simulink model "fizzbuzz"  (R2017a)
settings: Solver=VariableStepAuto  StartTime=0.0  StopTime=31.0  RelTol=1e-3
libraries: simulink x5, dspswit3 x1
settings Model: Creator=reyesc  LastModifiedBy=reyesc

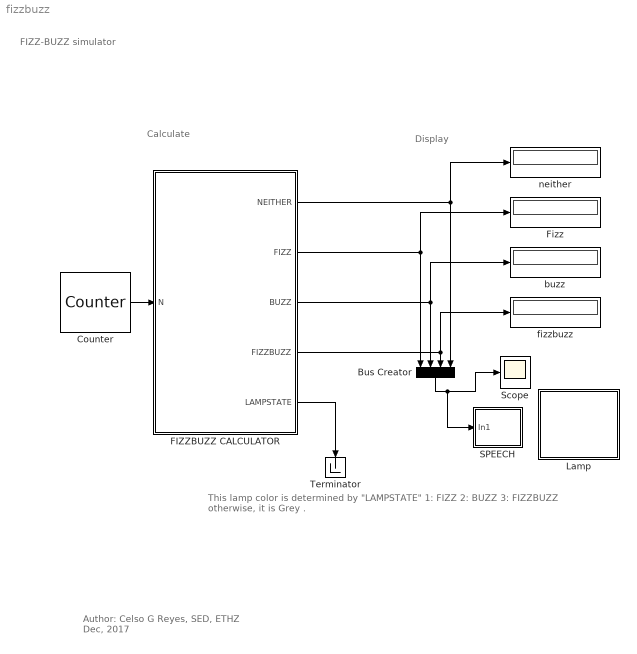
== system fizzbuzz ==
  note: Display
  note: Calculate
  note: This lamp color is determined by "LAMPSTATE"
      |
      | 1: FIZZ
      | 2: BUZZ
      | 3: FIZZBUZZ
      |
      | otherwise, it is Grey .
  note: Author: Celso G Reyes, SED, ETHZ
      | Dec, 2017
  note: FIZZ-BUZZ simulator
  Bus Creator : BusCreator  Inputs=4
  Counter : dspswit3/Counter  Direction=Up  CountEvent=Free running  CounterSize=User defined  MaxCount=100  InitialCount=0  Output=Count  HitValue=32  ResetInput=on  SamplesPerFrame=1  Ts=1  CntDtype=double  HitDtype=Logical
  FIZZBUZZ CALCULATOR : Subsystem
  Fizz : Display
  Lamp : Subsystem  DialogController=hmiCreateDDGDialog  IsWebBlock=on  mask(MWDashboardBlock){webBlockId=59f860f3-1faa-406f-b880-97fe9cd8e32d, webBlockType=lamp, ShowInLibBrowser=on, ShowInitialText=on, HMISrcModelName=fizzbuzz_simulator_c}
      mask prompts: webBlockType "WebBlock Type"; HMISrcModelName "Source Model"
      mask help: SimulinkHMI:dialogs:LampDialogDesc
      mask Help: helpview([docroot '/mapfiles/simulink.map'], 'hmi_lamp')
      mask Display:
      | if strcmp(get_param(bdroot(gcb),'BlockDiagramType'), 'library')
      |     image([(matlabroot) '/toolbox/simulink/hmi/icons/Lamp.png']);
      | end
  SPEECH : Subsystem
  Scope : Scope
  Terminator : Terminator
  buzz : Display
  fizzbuzz : Display
  neither : Display
  wires:
  Bus Creator/1 -> SPEECH/1(In1), Scope/1
  FIZZBUZZ CALCULATOR/4(FIZZBUZZ) -> fizzbuzz/1, Bus Creator/3
  FIZZBUZZ CALCULATOR/3(BUZZ) -> buzz/1, Bus Creator/2
  FIZZBUZZ CALCULATOR/2(FIZZ) -> Fizz/1, Bus Creator/1
  FIZZBUZZ CALCULATOR/1(NEITHER) -> neither/1, Bus Creator/4
  Counter/1 -> FIZZBUZZ CALCULATOR/1(N)
  FIZZBUZZ CALCULATOR/5(LAMPSTATE) -> Terminator/1

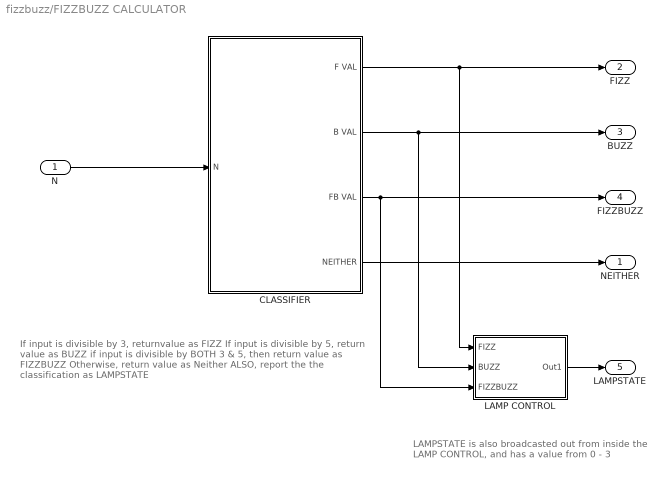
== system fizzbuzz/FIZZBUZZ CALCULATOR ==
  note: If input is divisible by 3, returnvalue as FIZZ
      |
      | If input is divisible by 5, return value as BUZZ
      |
      | if input is divisible by BOTH 3 & 5, then
      | return value as FIZZBUZZ
      |
      | Otherwise, return value as Neither
      |
      | ALSO, report the the classification as LAMPSTATE
  note: LAMPSTATE is also broadcasted out from inside
      | the LAMP CONTROL, and has a value from 0 - 3
  N : Inport
  CLASSIFIER : Subsystem
  LAMP CONTROL : Subsystem
  NEITHER : Outport
  FIZZ : Outport  Port=2
  BUZZ : Outport  Port=3
  FIZZBUZZ : Outport  Port=4
  LAMPSTATE : Outport  Port=5
  wires:
  LAMP CONTROL/1(Out1) -> LAMPSTATE/1
  N/1 -> CLASSIFIER/1(N)
  CLASSIFIER/4(NEITHER) -> NEITHER/1
  CLASSIFIER/3(FB VAL) -> LAMP CONTROL/3(FIZZBUZZ), FIZZBUZZ/1
  CLASSIFIER/1(F VAL) -> FIZZ/1, LAMP CONTROL/1(FIZZ)
  CLASSIFIER/2(B VAL) -> BUZZ/1, LAMP CONTROL/2(BUZZ)

== system fizzbuzz/Lamp ==

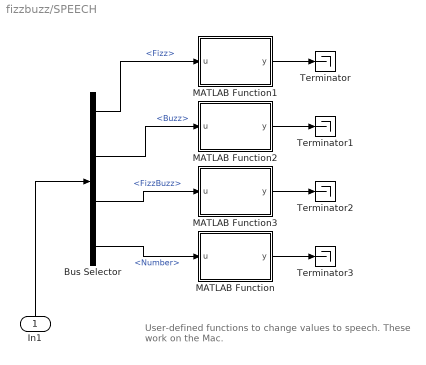
== system fizzbuzz/SPEECH ==
  note: User-defined functions to change values to speech.
      | These work on the Mac.
  In1 : Inport
  Bus Selector : BusSelector  OutputSignals=Fizz,Buzz,FizzBuzz,Number
  MATLAB Function : MATLAB Function  TreatAsAtomicUnit=on
  MATLAB Function1 : MATLAB Function  TreatAsAtomicUnit=on
  MATLAB Function2 : MATLAB Function  TreatAsAtomicUnit=on
  MATLAB Function3 : MATLAB Function  TreatAsAtomicUnit=on
  Terminator{,1..3} (4 alike) : Terminator
  wires:
  In1/1 -> Bus Selector/1
  Bus Selector/2 -> MATLAB Function2/1(u)  "<Buzz>"
  MATLAB Function2/1(y) -> Terminator1/1
  MATLAB Function3/1(y) -> Terminator2/1
  MATLAB Function1/1(y) -> Terminator/1
  Bus Selector/1 -> MATLAB Function1/1(u)  "<Fizz>"
  Bus Selector/4 -> MATLAB Function/1(u)  "<Number>"
  Bus Selector/3 -> MATLAB Function3/1(u)  "<FizzBuzz>"
  MATLAB Function/1(y) -> Terminator3/1

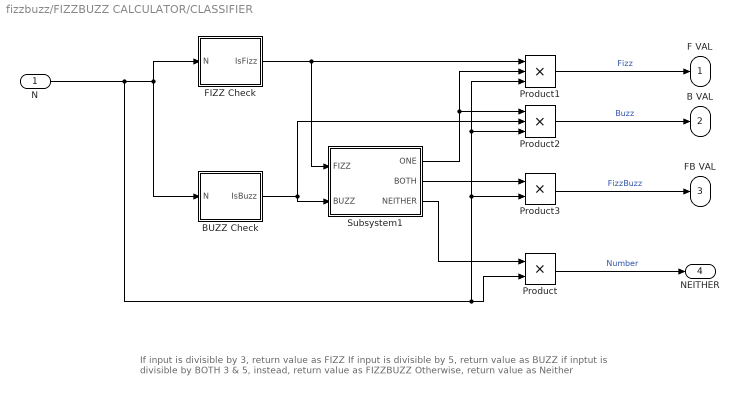
== system fizzbuzz/FIZZBUZZ CALCULATOR/CLASSIFIER ==
  note: If input is divisible by 3, return value as FIZZ
      | If input is divisible by 5, return value as BUZZ
      | if inptut is divisible by BOTH 3 & 5, instead, return value as FIZZBUZZ
      | Otherwise, return value as Neither
  N : Inport
  BUZZ Check : Subsystem
  FIZZ Check : Subsystem
  Product : Product
  Product1 : Product  Inputs=3
  Product2 : Product  Inputs=3
  Product3 : Product
  Subsystem1 : Subsystem
  F VAL : Outport
  B VAL : Outport  Port=2
  FB VAL : Outport  Port=3
  NEITHER : Outport  Port=4
  wires:
  Product1/1 -> F VAL/1  "Fizz"
  Product3/1 -> FB VAL/1  "FizzBuzz"
  Product/1 -> NEITHER/1  "Number"
  N/1 -> Product3/2, Product1/3, Product2/3, Product/2, BUZZ Check/1(N), FIZZ Check/1(N)
  Product2/1 -> B VAL/1  "Buzz"
  BUZZ Check/1(IsBuzz) -> Subsystem1/2(BUZZ), Product2/2
  FIZZ Check/1(IsFizz) -> Product1/1, Subsystem1/1(FIZZ)
  Subsystem1/2(BOTH) -> Product3/1
  Subsystem1/3(NEITHER) -> Product/1
  Subsystem1/1(ONE) -> Product1/2, Product2/1

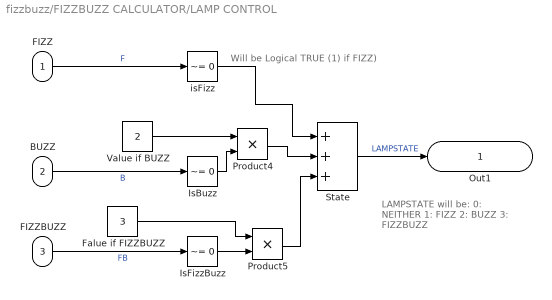
== system fizzbuzz/FIZZBUZZ CALCULATOR/LAMP CONTROL ==
  note: Will be Logical TRUE (1) if FIZZ)
  note: LAMPSTATE will be:
      |
      | 0: NEITHER
      | 1: FIZZ
      | 2: BUZZ
      | 3: FIZZBUZZ
  FIZZ : Inport
  BUZZ : Inport  Port=2
  FIZZBUZZ : Inport  Port=3
  Falue if FIZZBUZZ : Constant  Value=3
  IsBuzz : simulink/Logic and Bit Operations/Compare To Zero  relop=~=  OutDataTypeStr=boolean
  IsFizzBuzz : simulink/Logic and Bit Operations/Compare To Zero  relop=~=  OutDataTypeStr=boolean
  Product4 : Product
  Product5 : Product
  State : Sum  Inputs=+++
  Value if BUZZ : Constant  Value=2
  isFizz : simulink/Logic and Bit Operations/Compare To Zero  relop=~=  OutDataTypeStr=boolean
  Out1 : Outport
  wires:
  IsFizzBuzz/1 -> Product5/2
  isFizz/1 -> State/1
  Product4/1 -> State/2
  IsBuzz/1 -> Product4/2
  Product5/1 -> State/3
  Falue if FIZZBUZZ/1 -> Product5/1
  Value if BUZZ/1 -> Product4/1
  State/1 -> Out1/1  "LAMPSTATE"
  FIZZ/1 -> isFizz/1  "F"
  BUZZ/1 -> IsBuzz/1  "B"
  FIZZBUZZ/1 -> IsFizzBuzz/1  "FB"

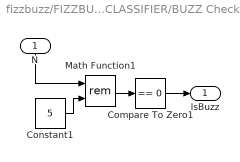
== system fizzbuzz/FIZZBUZZ CALCULATOR/CLASSIFIER/BUZZ Check ==
  N : Inport
  Compare To Zero1 : simulink/Logic and Bit Operations/Compare To Zero  relop===  OutDataTypeStr=boolean
  Constant1 : Constant  Value=5
  Math Function1 : Math  Operator=rem  SaturateOnIntegerOverflow=on
  IsBuzz : Outport
  wires:
  Constant1/1 -> Math Function1/2
  Math Function1/1 -> Compare To Zero1/1
  Compare To Zero1/1 -> IsBuzz/1
  N/1 -> Math Function1/1

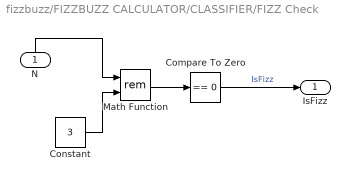
== system fizzbuzz/FIZZBUZZ CALCULATOR/CLASSIFIER/FIZZ Check ==
  N : Inport
  Compare To Zero : simulink/Logic and Bit Operations/Compare To Zero  relop===  OutDataTypeStr=boolean
  Constant : Constant  Value=3
  Math Function : Math  Operator=rem  SaturateOnIntegerOverflow=on
  IsFizz : Outport
  wires:
  Compare To Zero/1 -> IsFizz/1  "IsFizz"
  Math Function/1 -> Compare To Zero/1
  Constant/1 -> Math Function/2
  N/1 -> Math Function/1

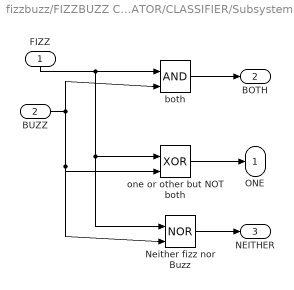
== system fizzbuzz/FIZZBUZZ CALCULATOR/CLASSIFIER/Subsystem1 ==
  FIZZ : Inport
  BUZZ : Inport  Port=2
  Neither fizz nor Buzz : Logic  Operator=NOR  IconShape=distinctive  AllPortsSameDT=off  OutDataTypeStr=boolean
  both : Logic  IconShape=distinctive  AllPortsSameDT=off  OutDataTypeStr=boolean
  one or other but NOT both : Logic  Operator=XOR  IconShape=distinctive  AllPortsSameDT=off  OutDataTypeStr=boolean
  ONE : Outport
  BOTH : Outport  Port=2
  NEITHER : Outport  Port=3
  wires:
  Neither fizz nor Buzz/1 -> NEITHER/1
  both/1 -> BOTH/1
  one or other but NOT both/1 -> ONE/1
  BUZZ/1 -> one or other but NOT both/2, Neither fizz nor Buzz/2, both/2
  FIZZ/1 -> one or other but NOT both/1, Neither fizz nor Buzz/1, both/1

== matlab function fizzbuzz/SPEECH/MATLAB Function1 ==
  data: u input; y output
function y = sayFizz(u)
    coder.extrinsic('system')
    if u ~= 0
        cmd=['say "fizz"'];
        system(cmd)
    end
    y = u;
end

== matlab function fizzbuzz/SPEECH/MATLAB Function ==
  data: u input; y output
function y = sayNumber(u)
    coder.extrinsic('system')
    coder.extrinsic('sprintf')
    if u ~= 0
        cmd=['say ' sprintf('%d',u)];
        system(cmd)
    end
    y = u;
end

== matlab function fizzbuzz/SPEECH/MATLAB Function2 ==
  data: u input; y output
function y = sayBuzz(u)
    coder.extrinsic('system')
    if u ~= 0
        cmd=['say "buzz"'];
        system(cmd)
    end
    y = u;
end

== matlab function fizzbuzz/SPEECH/MATLAB Function3 ==
  data: u input; y output
function y = sayFizzBuzz(u)
    coder.extrinsic('system')
    if u ~= 0
        cmd=['say "fizzbuzz"'];
        system(cmd)
    end
    y = u;
end
